simulink model "Laengsdynamikmodell_NEmo_MonteCarlo_TestBench"  (R2020b)
settings: Solver=FixedStepAuto  StartTime=0.0  StopTime=1477  FixedStep=0.01  RelTol=1e-3
model workspace (MAT data in the model file):
  C_RR = 0.0103682470085
  SampleTime = 0.01
  StopTime = 1477
  UncertaintyRollerDynamometer = 0.796984855506
  VehMass = 929
  c_w = 0.37
  cycle = timeseries
  cycle.Name = 'VehSpeed'
  cycle.DataInfo = tsdata.datametadata
  cycle.DataInfo.Interpolation = tsdata.interpolation
  cycle.DataInfo.Interpolation.Fhandle : function handle (value not decoded)
  cycle.DataInfo.Interpolation.Name = 'linear'
  cycle.TimeInfo = tsdata.timemetadata
  cycle.TimeInfo.Length = 147701
  cycle.TimeInfo.DuplicateTimes = 0
  cycle.TimeInfo.Increment_ = 0.01
  cycle.TimeInfo.Start_ = 0
  cycle.TimeInfo.Initialized = 1
  cycle.QualityInfo = tsdata.qualmetadata
  cycle.Data_ = [0.00117951013636 0.00115673379699 0.00113506916288 0.00111379623058 0.00109291828727 0.00107244937706 0.00105240927603 0.00103281507454 0.00101368170682 0.000995077988387 0.000977002820608 0.000959146553684 ... (147701 elements, 147701x1)]
  i_gear = 5.6813
  p = 2.5
  power_map_LE = [81.3594367777 81.3594367777 88.9151238368 69.3920543425 121.856227925 33.5913037104 56.5214963128 60.6342218487 61.1595876762 53.4292335319 53.4133899816 35.6771556802 ... (16260 elements, 60x271)]
  power_map_Mot = [0 74.834999341 40.2428359465 95.3690451807 75.6091573236 114.707467852 143.074401876 144.922747771 177.284289075 184.351766643 192.404587732 197.413952644 ... (16260 elements, 60x271)]
  r_dyn = 0.275233869952
undefined symbols (not defined in the file): DiscIntNeverNeededParam, gravity, UncertaintyMappedLosses, UncertaintyTabledConsumption, v_HA
libraries: Constant_Environment x1, Driver_PI x1, Longitudinal_DrivingCycles x1, Acceleration_Calculation x1, Air_Resistance x1, Roll_Resistance x1, Slope_Resistance x1, Simple_Auxiliary x1, Electric_Drive_Tabled_Consumption x1, Gear_Stage x1, DCAC_Converter x1, Control_Unit_Simple x1
(part 1 of 3)
settings Model: SimulationMode=accelerator  NumberOfSteps=1000  OrderedModelArguments=off  Creator=Tony  LastModifiedBy=ga69qig
settings DataIOCC: ReturnWorkspaceOutputs=off
settings DebuggingCC: ArithmeticOperatorsInVariantConditions=warning
settings SFSimCC: SimUseLocalCustomCode=off  CustomCodeUndefinedFunction=UseInterfaceOnly
settings RTWCC: RTWUseLocalCustomCode=off
settings CodeAppCC: StateflowObjectComments=on

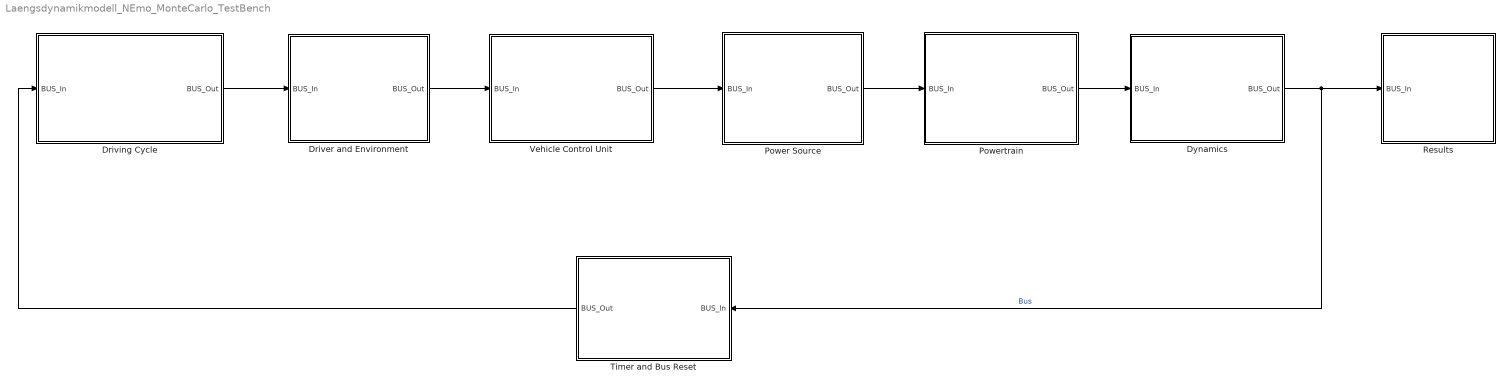
== system Laengsdynamikmodell_NEmo_MonteCarlo_TestBench ==
  Driver and Environment : Subsystem
      mask help:
      | <Author> Alexander Koch based on Stefan Müller, Stephan Rohr
      | <Date> 03/04/2017
      |
      | <Description>
      | Consist of a Bus In and a Bus Out Block. To Select Signals from the Bus open the Bus In Block, to write signals to the Bus under a certain tab name open the bus out block. For further information, please read the discription of the Bus In and Bus out Block
      |
      | The Block automaticlly disconnects the link to the library block after opening the first time
      |
      | <Parameters>
      | -
      |
      | <Inputs>
      | BUS_In [Bus]
      |
      | <Outputs>
      | Bus_Out [Bus]
      settings: OpenFcn=|
      | set_param(gcb(),'LinkStatus','none')
      | open_system(gcb(),'force')
      mask Display:
      | [picturexpos,pictureypos,picturewidth,pictureheight] = ...
      |     CalcBlockPicturePosition(gcb,1,0.01,0.1,30,30); % calculating picture position depending on Block size and minimum margin size
      | image('Driver_PI.svg',[picturexpos pictureypos picturewidth pictureheight]); % plot picture to block
  Driving Cycle : Subsystem
      mask help:
      | <Author> Alexander Koch based on Stefan Müller, Stephan Rohr
      | <Date> 03/04/2017
      |
      | <Description>
      | Consist of a Bus In and a Bus Out Block. To Select Signals from the Bus open the Bus In Block, to write signals to the Bus under a certain tab name open the bus out block. For further information, please read the discription of the Bus In and Bus out Block
      |
      | The Block automaticlly disconnects the link to the library block after opening the first time
      |
      | <Parameters>
      | -
      |
      | <Inputs>
      | BUS_In [Bus]
      |
      | <Outputs>
      | Bus_Out [Bus]
      settings: OpenFcn=|
      | set_param(gcb(),'LinkStatus','none')
      | open_system(gcb(),'force')
      mask Display:
      | [picturexpos,pictureypos,picturewidth,pictureheight] = ...
      |     CalcBlockPicturePosition(gcb,1,0.01,0.1,50,50); % calculating picture position depending on Block size and minimum margin size
      | image('Longitudinal_DrivingCycles.svg',[picturexpos pictureypos picturewidth pictureheight]); % plot picture to block
  Dynamics : Subsystem
      mask help:
      | <Author> Alexander Koch based on Stefan Müller, Stephan Rohr
      | <Date> 03/04/2017
      |
      | <Description>
      | Consist of a Bus In and a Bus Out Block. To Select Signals from the Bus open the Bus In Block, to write signals to the Bus under a certain tab name open the bus out block. For further information, please read the discription of the Bus In and Bus out Block
      |
      | The Block automaticlly disconnects the link to the library block after opening the first time
      |
      | <Parameters>
      | -
      |
      | <Inputs>
      | BUS_In [Bus]
      |
      | <Outputs>
      | Bus_Out [Bus]
      settings: OpenFcn=|
      | set_param(gcb(),'LinkStatus','none')
      | open_system(gcb(),'force')
      mask Display:
      | [picturexpos,pictureypos,picturewidth,pictureheight] = ...
      |     CalcBlockPicturePosition(gcb,1,0.01,0.1,40,50); % calculating picture position depending on Block size and minimum margin size
      | image('Acceleration_Calculation.svg',[picturexpos pictureypos picturewidth pictureheight]); % plot picture to block
  Power Source : Subsystem
      mask help:
      | <Author> Alexander Koch based on Stefan Müller, Stephan Rohr
      | <Date> 03/04/2017
      |
      | <Description>
      | Consist of a Bus In and a Bus Out Block. To Select Signals from the Bus open the Bus In Block, to write signals to the Bus under a certain tab name open the bus out block. For further information, please read the discription of the Bus In and Bus out Block
      |
      | The Block automaticlly disconnects the link to the library block after opening the first time
      |
      | <Parameters>
      | -
      |
      | <Inputs>
      | BUS_In [Bus]
      |
      | <Outputs>
      | Bus_Out [Bus]
      settings: OpenFcn=|
      | set_param(gcb(),'LinkStatus','none')
      | open_system(gcb(),'force')
      mask Display:
      | [picturexpos,pictureypos,picturewidth,pictureheight] = ...
      |     CalcBlockPicturePosition(gcb,3/6,0.01,0.1,40,40); % calculating picture position depending on Block size and minimum margin size
      | image('Constant_Power_Source.svg',[picturexpos pictureypos picturewidth pictureheight]); % plot picture to block
  Powertrain : Subsystem
      mask help:
      | <Author> Alexander Koch based on Stefan Müller, Stephan Rohr
      | <Date> 03/04/2017
      |
      | <Description>
      | Consist of a Bus In and a Bus Out Block. To Select Signals from the Bus open the Bus In Block, to write signals to the Bus under a certain tab name open the bus out block. For further information, please read the discription of the Bus In and Bus out Block
      |
      | The Block automaticlly disconnects the link to the library block after opening the first time
      |
      | <Parameters>
      | -
      |
      | <Inputs>
      | BUS_In [Bus]
      |
      | <Outputs>
      | Bus_Out [Bus]
      settings: OpenFcn=|
      | set_param(gcb(),'LinkStatus','none')
      | open_system(gcb(),'force')
      mask Display:
      | [picturexpos,pictureypos,picturewidth,pictureheight] = ...
      |     CalcBlockPicturePosition(gcb,1,0.01,0.1,40,40); % calculating picture position depending on Block size and minimum margin size
      | image('Electric_Drive_Simple_Efficiency.svg',[picturexpos pictureypos picturewidth pictureheight]); % plot picture to block
  Results : Subsystem
      mask help:
      | <Author> Alexander Koch
      | <Date> 03/04/2017
      | <Predecessor> Stefan Müller, Stephan Rohr
      |
      | <Description>
      | Consist of a Bus In and a Bus Out Block. To Select Signals from the Bus open the Bus In Block, to write signals to the Bus under a certain tab name open the bus out block. For further information, please read the discription of the Bus In and Bus out Block
      |
      | The Block automaticlly disconnects the link to the library block after opening the first time
      |
      | <Parameters>
      | -
      |
      | <Inputs>
      | Bus [Bus]
      |
      | <Outputs>
      | Bus [Bus]
      settings: OpenFcn=|
      | set_param(gcb(),'LinkStatus','none')
      | open_system(gcb(),'force')
      mask Display:
      | [picturexpos,pictureypos,picturewidth,pictureheight] = ...
      |     CalcBlockPicturePosition(gcb,1,0.01,0.1,40,10); % calculating picture position depending on Block size and minimum margin size
      | image('Scopes_Simulation.svg',[picturexpos pictureypos picturewidth pictureheight]); % plot picture to block
  Timer and Bus Reset : Subsystem
      settings: OpenFcn=|
      | set_param(gcb(),'LinkStatus','none')
      | open_system(gcb(),'mask')
      mask DialogControl RefreshBus Prompt: Refresh Bus
      mask DialogControl RefreshBus Callback: TimerandBusResetRefreshBus()
      mask Display:
      | [picturexpos,pictureypos,picturewidth,pictureheight] = ...
      |     CalcBlockPicturePosition(gcb,1,0.01,0.1,50,50); % calculating picture position depending on Block size and minimum margin size
      | image('reset.png',[picturexpos pictureypos picturewidth pictureheight]); % plot picture to block
  Vehicle Control Unit : Subsystem
      mask help:
      | <Author> Alexander Koch based on Stefan Müller, Stephan Rohr
      | <Date> 03/04/2017
      |
      | <Description>
      | Consist of a Bus In and a Bus Out Block. To Select Signals from the Bus open the Bus In Block, to write signals to the Bus under a certain tab name open the bus out block. For further information, please read the discription of the Bus In and Bus out Block
      |
      | The Block automaticlly disconnects the link to the library block after opening the first time
      |
      | <Parameters>
      | -
      |
      | <Inputs>
      | BUS_In [Bus]
      |
      | <Outputs>
      | Bus_Out [Bus]
      settings: OpenFcn=|
      | set_param(gcb(),'LinkStatus','none')
      | open_system(gcb(),'force')
      mask Display:
      | [picturexpos,pictureypos,picturewidth,pictureheight] = ...
      |     CalcBlockPicturePosition(gcb,1,0.01,0.1,30,30); % calculating picture position depending on Block size and minimum margin size
      | image('Control_Unit_Simple.svg',[picturexpos pictureypos picturewidth pictureheight]); % plot picture to block
  wires:
  Power Source/1(BUS_Out) -> Powertrain/1(BUS_In)
  Driver and Environment/1(BUS_Out) -> Vehicle Control Unit/1(BUS_In)
  Driving Cycle/1(BUS_Out) -> Driver and Environment/1(BUS_In)
  Vehicle Control Unit/1(BUS_Out) -> Power Source/1(BUS_In)
  Timer and Bus Reset/1(BUS_Out) -> Driving Cycle/1(BUS_In)
  Dynamics/1(BUS_Out) -> Timer and Bus Reset/1(BUS_In), Results/1(BUS_In)  "Bus"
  Powertrain/1(BUS_Out) -> Dynamics/1(BUS_In)
